simulink subsystem "SubsistemaMotores"  (R2022b)
settings: Solver=VariableStepAuto  StartTime=0.0  StopTime=10.0  RelTol=1e-3
libraries: arduinolib x6, simulink x2
settings Model: Creator=Usuario_UMA  LastModifiedBy=Usuario
settings OptimizationCC: ReuseModelBlockBuffer=on

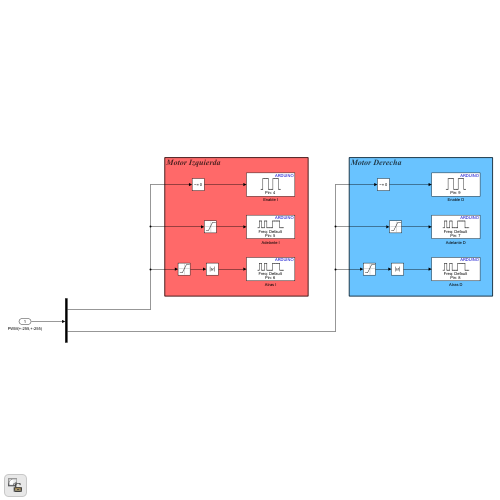
[thumbnail: Simulink's stored preview of the top-level diagram]
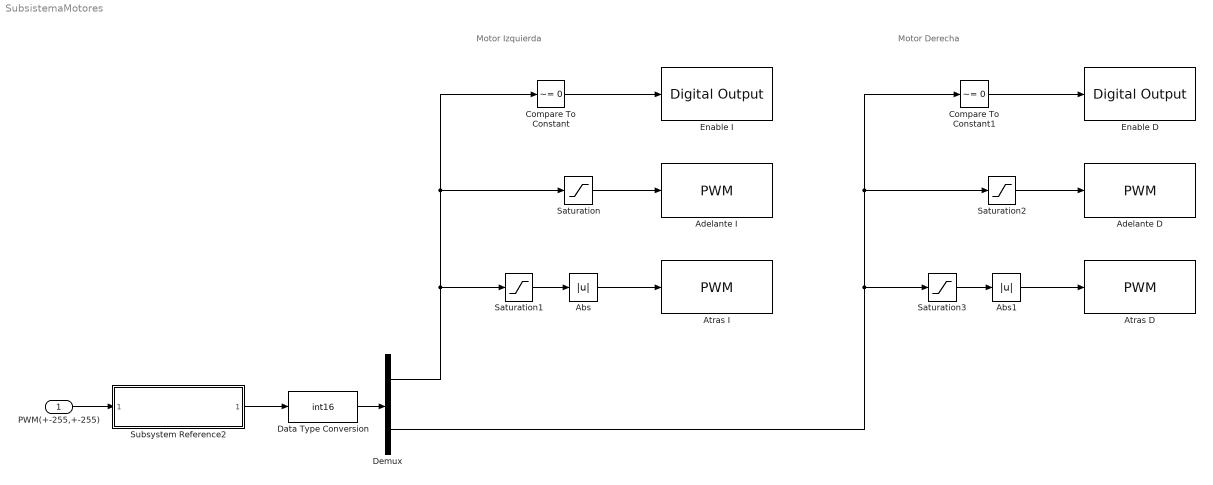
== system SubsistemaMotores ==
  note: Motor Izquierda
  note: Motor Derecha
  PWM(+-255,+-255) : Inport
  Abs : Abs  SaturateOnIntegerOverflow=off
  Abs1 : Abs  SaturateOnIntegerOverflow=off
  Adelante D : arduinolib/PWM  pinNumber=7  frequencyType=Default  desiredFrequency=490.2  achievableFrequency=490.2
  Adelante I : arduinolib/PWM  pinNumber=5  frequencyType=Default  desiredFrequency=490.2  achievableFrequency=490.2
  Atras D : arduinolib/PWM  pinNumber=8  frequencyType=Default  desiredFrequency=490.2  achievableFrequency=490.2
  Atras I : arduinolib/PWM  pinNumber=6  frequencyType=Default  desiredFrequency=490.2  achievableFrequency=490.2
  Compare To Constant : simulink/Logic and Bit Operations/Compare To Constant  relop=~=  const=0  OutDataTypeStr=boolean
  Compare To Constant1 : simulink/Logic and Bit Operations/Compare To Constant  relop=~=  const=0  OutDataTypeStr=boolean
  Data Type Conversion : DataTypeConversion  OutDataTypeStr=int16  SaturateOnIntegerOverflow=off  RndMeth=Floor
  Demux : Demux  Outputs=2
  Enable D : arduinolib/Digital Output  pinNumber=9  Direction=output  blockPlatform=arduino
  Enable I : arduinolib/Digital Output  pinNumber=4  Direction=output  blockPlatform=arduino
  Saturation : Saturate  UpperLimit=255  LowerLimit=1
  Saturation1 : Saturate  UpperLimit=0  LowerLimit=-255
  Saturation2 : Saturate  UpperLimit=255  LowerLimit=1
  Saturation3 : Saturate  UpperLimit=0  LowerLimit=-255
  Subsystem Reference2 : Subsystem  ReferencedSubsystem=MyPieroAjusteRuedas
  wires:
  PWM(+-255,+-255)/1 -> Subsystem Reference2/1
  Data Type Conversion/1 -> Demux/1
  Subsystem Reference2/1 -> Data Type Conversion/1
  Compare To Constant/1 -> Enable I/1
  Saturation/1 -> Adelante I/1
  Saturation1/1 -> Abs/1
  Abs/1 -> Atras I/1
  Saturation2/1 -> Adelante D/1
  Abs1/1 -> Atras D/1
  Saturation3/1 -> Abs1/1
  Compare To Constant1/1 -> Enable D/1
  Demux/1 -> Saturation1/1, Compare To Constant/1, Saturation/1
  Demux/2 -> Saturation3/1, Compare To Constant1/1, Saturation2/1
